simulink model "Sub_1"  (R2018a)
settings: Solver=VariableStepAuto  StartTime=0.0  StopTime=10.0  RelTol=1e-3
settings Model: Creator=midog  LastModifiedBy=midog

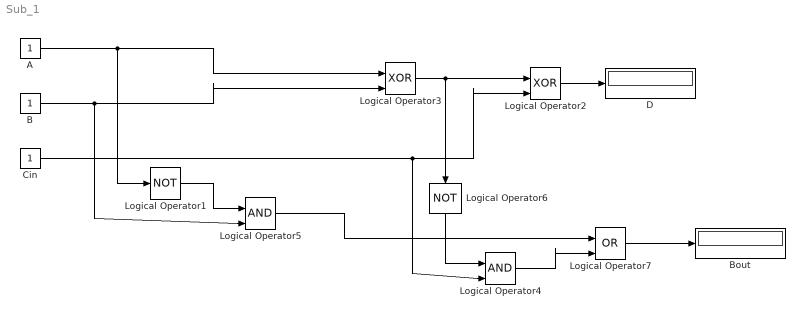
== system Sub_1 ==
  A : Constant
  B : Constant
  Bout : Display
  Cin : Constant
  D : Display
  Logical Operator1 : Logic  Operator=NOT  IconShape=distinctive  AllPortsSameDT=off  OutDataTypeStr=boolean
  Logical Operator2 : Logic  Operator=XOR  IconShape=distinctive  AllPortsSameDT=off  OutDataTypeStr=boolean
  Logical Operator3 : Logic  Operator=XOR  IconShape=distinctive  AllPortsSameDT=off  OutDataTypeStr=boolean
  Logical Operator4 : Logic  IconShape=distinctive  AllPortsSameDT=off  OutDataTypeStr=boolean
  Logical Operator5 : Logic  IconShape=distinctive  AllPortsSameDT=off  OutDataTypeStr=boolean
  Logical Operator6 : Logic  Operator=NOT  IconShape=distinctive  AllPortsSameDT=off  OutDataTypeStr=boolean
  Logical Operator7 : Logic  Operator=OR  IconShape=distinctive  AllPortsSameDT=off  OutDataTypeStr=boolean
  wires:
  Logical Operator2/1 -> D/1
  Logical Operator3/1 -> Logical Operator6/1, Logical Operator2/1
  B/1 -> Logical Operator5/2, Logical Operator3/2
  A/1 -> Logical Operator1/1, Logical Operator3/1
  Logical Operator1/1 -> Logical Operator5/1
  Cin/1 -> Logical Operator4/2, Logical Operator2/2
  Logical Operator6/1 -> Logical Operator4/1
  Logical Operator5/1 -> Logical Operator7/1
  Logical Operator4/1 -> Logical Operator7/2
  Logical Operator7/1 -> Bout/1
